simulink model "at_slk_HBA"  (R2017b)
settings: Solver=FixedStepDiscrete  StartTime=0.0  StopTime=10.0  FixedStep=1  RelTol=1e-3
PreLoadFcn:
  | sl_refresh_customizations
  | enum_Simulink
  | simulinkExportUnitCs
  | E_Global_Constants
  | A_Data_Dictionary
  | 
  | bus_Simulink
InitFcn:
  | checkUnitMismatch
model workspace (MAT data in the model file):
  ESD_URL = 'http://127.0.0.1:63320/node?ref=r%3A92f02917-2939-4625-878a-0cf4bf3cdc0b%28AHCDemo._30_Implementation%29%2F458597115437889651'
undefined symbols (not defined in the file): eBeamState, Global_Constants
libraries: simulink x4
settings Model: Creator=ohm9xd  LastModifiedBy=eh6qym
settings OptimizationCC: DefaultParameterBehavior=Inlined  PassReuseOutputArgsAs=Individual arguments  ZeroExternalMemoryAtStartup=off
settings DebuggingCC: SignalRangeChecking=error  InheritedTsInSrcMsg=none  ParameterTunabilityLossMsg=error
settings SFSimCC: MATLABDynamicMemAlloc=off
settings RTWCC: SystemTargetFile=esd_ert.tlc  GenCodeOnly=on  TemplateMakefile=ert_default_tmf  Description=CSD  GenerateReport=on  IncludeHyperlinkInReport=on  LaunchReport=on  GenerateTraceInfo=on  GenerateTraceReport=on  GenerateTraceReportSl=on  GenerateTraceReportSf=on  GenerateTraceReportEml=on
settings CodeAppCC: ForceParamTrailComments=on  IgnoreCustomStorageClasses=off  OperatorAnnotations=on  SimulinkDataObjDesc=on  SFDataObjDesc=on  InsertBlockDesc=on
settings STFCustomTargetCC: TargetLangStandard=C99 (ISO)  MultiwordLength=256  GenerateSampleERTMain=on  IncludeMdlTerminateFcn=off  CombineOutputUpdateFcns=on  CombineSignalStateStructs=on  SuppressErrorStatus=on  ERTCustomFileBanners=on  MultiInstanceERTCode=on  CodeInterfacePackaging=Reusable function  SupportContinuousTime=off  SupportNonInlinedSFcns=off  RemoveDisableFunc=on  RemoveResetFunc=on  MATLABClassNameForMDSCustomization=Simulink.SoftwareTarget.ERTCustomization  GRTInterface=off  SystemTargetFile=esd_ert.tlc
settings ERTTargetCC: TargetLangStandard=C99 (ISO)  GenerateSampleERTMain=on  ParMdlRefBuildCompliant=off  CompOptLevelCompliant=off  ConcurrentExecutionCompliant=off  IncludeMdlTerminateFcn=off  CombineSignalStateStructs=on  SuppressErrorStatus=on  MultiInstanceERTCode=on  CodeInterfacePackaging=Reusable function  RemoveDisableFunc=on  ModelStepFunctionPrototypeControlCompliant=off  CPPClassGenCompliant=off  UseToolchainInfoCompliant=off  InlinedParameterPlacement=NonHierarchical  ERTCustomFileTemplate=example_file_process.tlc

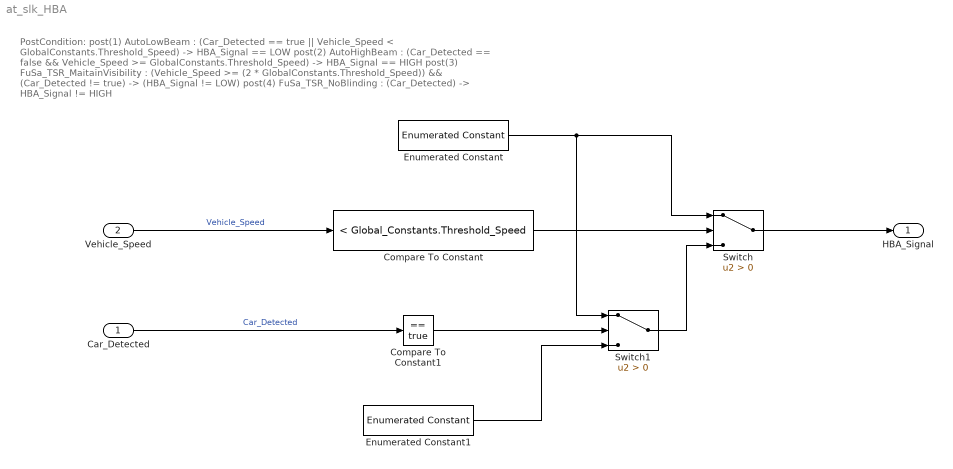
== system at_slk_HBA ==
  note: PostCondition:
      | post(1) AutoLowBeam :   (Car_Detected == true || Vehicle_Speed < GlobalConstants.Threshold_Speed) -> HBA_Signal == LOW
      | post(2) AutoHighBeam :   (Car_Detected == false && Vehicle_Speed >= GlobalConstants.Threshold_Speed) -> HBA_Signal == HIGH
      | post(3) FuSa_TSR_MaitainVisibility :   (Vehicle_Speed >= (2 * GlobalConstants.Threshold_Speed)) && (Car_Detected != true) -> (HBA_Signal != LOW)
      | post(4) FuSa_TSR_NoBlinding :   (Car_Detected) -> HBA_Signal != HIGH
  Car_Detected : Inport  OutDataTypeStr=boolean
  Vehicle_Speed : Inport  Port=2  OutDataTypeStr=double  Unit=kmph
      settings: AttributesFormatString=(kmph)
  Compare To Constant : simulink/Logic and Bit Operations/Compare To Constant  relop=<  const=Global_Constants.Threshold_Speed  OutDataTypeStr=boolean
  Compare To Constant1 : simulink/Logic and Bit Operations/Compare To Constant  relop===  const=true  OutDataTypeStr=boolean
  Enumerated Constant : simulink/Sources/Enumerated Constant  OutDataTypeStr=Enum: eBeamState  Value=eBeamState.LOW  SampleTime=inf
      settings: SourceProductName=Simulink
  Enumerated Constant1 : simulink/Sources/Enumerated Constant  OutDataTypeStr=Enum: eBeamState  Value=eBeamState.HIGH  SampleTime=inf
      settings: SourceProductName=Simulink
  Switch : Switch  Criteria=u2 > Threshold
  Switch1 : Switch  Criteria=u2 > Threshold
  HBA_Signal : Outport  OutDataTypeStr=Enum: eBeamState_t
  wires:
  Vehicle_Speed/1 -> Compare To Constant/1  "Vehicle_Speed"
  Compare To Constant/1 -> Switch/2
  Enumerated Constant/1 -> Switch1/1, Switch/1
  Switch/1 -> HBA_Signal/1
  Car_Detected/1 -> Compare To Constant1/1  "Car_Detected"
  Compare To Constant1/1 -> Switch1/2
  Switch1/1 -> Switch/3
  Enumerated Constant1/1 -> Switch1/3
